simulink model "simDron"  (R2024a)
settings: Solver=VariableStepAuto  StartTime=0.0  StopTime=t  RelTol=1e-6  AbsTol=1e-9
values from neighbouring files (symbols this model uses):
  d0 = [0;0;-2]    [Dron.m]
  I = [Ixx, 0, 0 ... (first row only)    [Dron.m]
  Jr = -5.897e-8    (= -5.897e-08)    [Dron.m]
  km = 803.9    [Dron.m]
  KQ = 1.058e-10    [Dron.m]
  KT = 3.334e-8    (= 3.334e-08)    [Dron.m]
  l = 0.058    [Dron.m]
  m = 0.045    [Dron.m]
  mg = [0;0;m*9.81]    [Dron.m]
  theta0 = [0;0;0]    [Dron.m]
  u1 = 10000    [Dron.m]
  u2 = 5000    [Dron.m]
  u3 = 10000    [Dron.m]
  u4 = 5000    [Dron.m]
  v0 = [0;0;0]    [Dron.m]
  w0 = [0;0;0]    [Dron.m]
libraries: matrix_library x2
settings Model: Creator=oscka  LastModifiedBy=oscka
settings DataIOCC: SaveOutput=off  SignalLogging=off  DSMLogging=off  SaveTime=off  ReturnWorkspaceOutputs=off

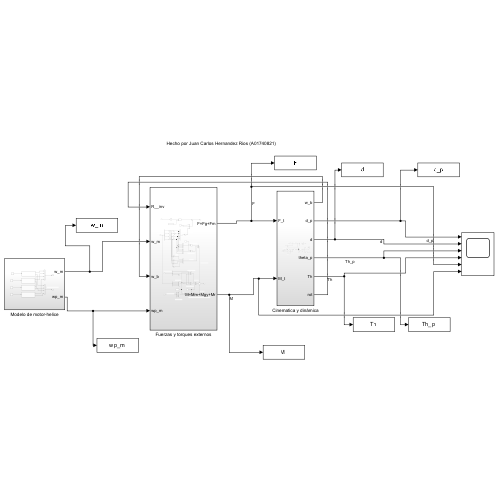
[thumbnail: Simulink's stored preview of the top-level diagram]
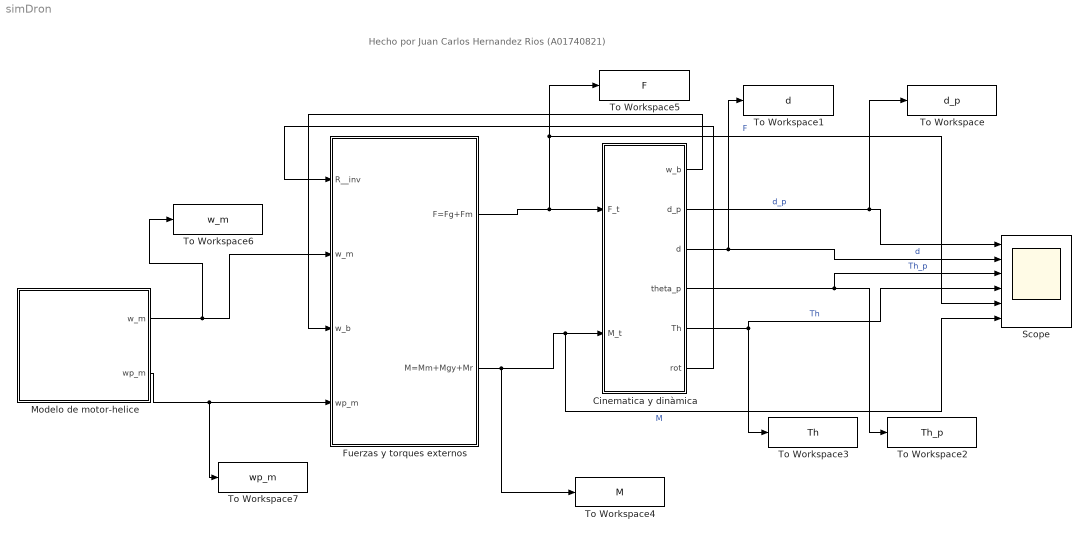
== system simDron ==
  note: Hecho por Juan Carlos Hernandez Rios (A01740821)
  Cinematica y dinàmica : Subsystem
  Fuerzas y torques externos : Subsystem
  Modelo de motor-helice : Subsystem
  Scope : Scope  NumInputPorts=6
  To Workspace : ToWorkspace  VariableName=d_p  SaveFormat=Timeseries  SampleTime=-1
  To Workspace1 : ToWorkspace  VariableName=d  SaveFormat=Timeseries  SampleTime=-1
  To Workspace2 : ToWorkspace  VariableName=Th_p  SaveFormat=Timeseries  SampleTime=-1
  To Workspace3 : ToWorkspace  VariableName=Th  SaveFormat=Timeseries  SampleTime=-1
  To Workspace4 : ToWorkspace  VariableName=M  SaveFormat=Timeseries  SampleTime=-1
  To Workspace5 : ToWorkspace  VariableName=F  SaveFormat=Timeseries  SampleTime=-1
  To Workspace6 : ToWorkspace  VariableName=w_m  SaveFormat=Timeseries  SampleTime=-1
  To Workspace7 : ToWorkspace  VariableName=wp_m  SaveFormat=Timeseries  SampleTime=-1
  wires:
  Modelo de motor-helice/1(w_m) -> To Workspace6/1, Fuerzas y torques externos/2(w_m)
  Modelo de motor-helice/2(wp_m) -> To Workspace7/1, Fuerzas y torques externos/4(wp_m)
  Fuerzas y torques externos/1(F=Fg+Fm) -> To Workspace5/1, Scope/5, Cinematica y dinàmica/1(F_t)  "F"
  Fuerzas y torques externos/2(M=Mm+Mgy+Mr) -> Scope/6, Cinematica y dinàmica/2(M_t), To Workspace4/1  "M"
  Cinematica y dinàmica/1(w_b) -> Fuerzas y torques externos/3(w_b)
  Cinematica y dinàmica/6(rot) -> Fuerzas y torques externos/1(R__inv)
  Cinematica y dinàmica/2(d_p) -> To Workspace/1, Scope/1  "d_p"
  Cinematica y dinàmica/3(d) -> Scope/2, To Workspace1/1  "d"
  Cinematica y dinàmica/4(theta_p) -> Scope/3, To Workspace2/1  "Th_p"
  Cinematica y dinàmica/5(Th) -> Scope/4, To Workspace3/1  "Th"

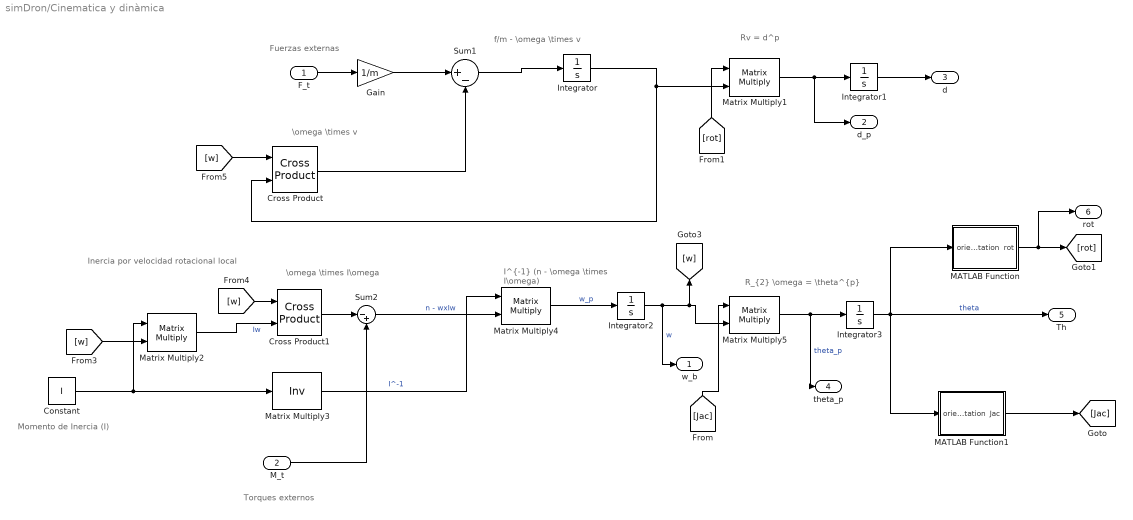
== system simDron/Cinematica y dinàmica ==
  note: Fuerzas externas
  note: Torques externos
  note: Rv = d^p
  note: \omega \times v
  note: f/m - \omega \times v
  note: I^{-1} (n - \omega \times I\omega)
  note: R_{2} \omega = \theta^{p}
  note: \omega \times I\omega
  note: Momento de Inercia (I)
  note: Inercia por velocidad rotacional local
  F_t : Inport
  M_t : Inport  Port=2
  Constant : Constant  Value=I  VectorParams1D=off
  Cross Product : matrix_library/Cross Product
  Cross Product1 : matrix_library/Cross Product
  Gain : Gain  Gain=1/m
  Integrator : Integrator  InitialCondition=v0
  Integrator1 : Integrator  InitialCondition=d0
  Integrator2 : Integrator  InitialCondition=w0
  Integrator3 : Integrator  InitialCondition=theta0
  MATLAB Function : MATLAB Function  TreatAsAtomicUnit=on
  MATLAB Function1 : MATLAB Function  TreatAsAtomicUnit=on
  Matrix Multiply{1..2,4..5} (4 alike) : Product  Multiplication=Matrix(*)
  Matrix Multiply3 : Product  Inputs=/  Multiplication=Matrix(*)
  Sum1 : Sum  Inputs=|+-
  Sum2 : Sum  Inputs=|-+
  w_b : Outport
  d_p : Outport  Port=2
  d : Outport  Port=3
  theta_p : Outport  Port=4
  Th : Outport  Port=5
  rot : Outport  Port=6
  wires:
  [Jac] -> Matrix Multiply5/1
  Matrix Multiply2/1 -> Cross Product1/2  "Iw"
  [w] -> Cross Product1/1
  [w] -> Matrix Multiply2/2
  MATLAB Function1/1(Jac) -> [Jac]
  Matrix Multiply1/1 -> d_p/1, Integrator1/1
  [w] -> Cross Product/1
  Matrix Multiply5/1 -> theta_p/1, Integrator3/1  "theta_p"
  Integrator2/1 -> w_b/1, [w], Matrix Multiply5/2  "w"
  Cross Product/1 -> Sum1/2
  Cross Product1/1 -> Sum2/1
  MATLAB Function/1(rot) -> rot/1, [rot]
  Matrix Multiply3/1 -> Matrix Multiply4/1  "I^-1"
  Matrix Multiply4/1 -> Integrator2/1  "w_p"
  Integrator3/1 -> MATLAB Function/1(orientation), MATLAB Function1/1(orientation), Th/1  "theta"
  Sum2/1 -> Matrix Multiply4/2  "n - wxIw"
  Constant/1 -> Matrix Multiply2/1, Matrix Multiply3/1
  Integrator/1 -> Matrix Multiply1/2, Cross Product/2
  [rot] -> Matrix Multiply1/1
  Sum1/1 -> Integrator/1
  Integrator1/1 -> d/1
  M_t/1 -> Sum2/2
  Gain/1 -> Sum1/1
  F_t/1 -> Gain/1

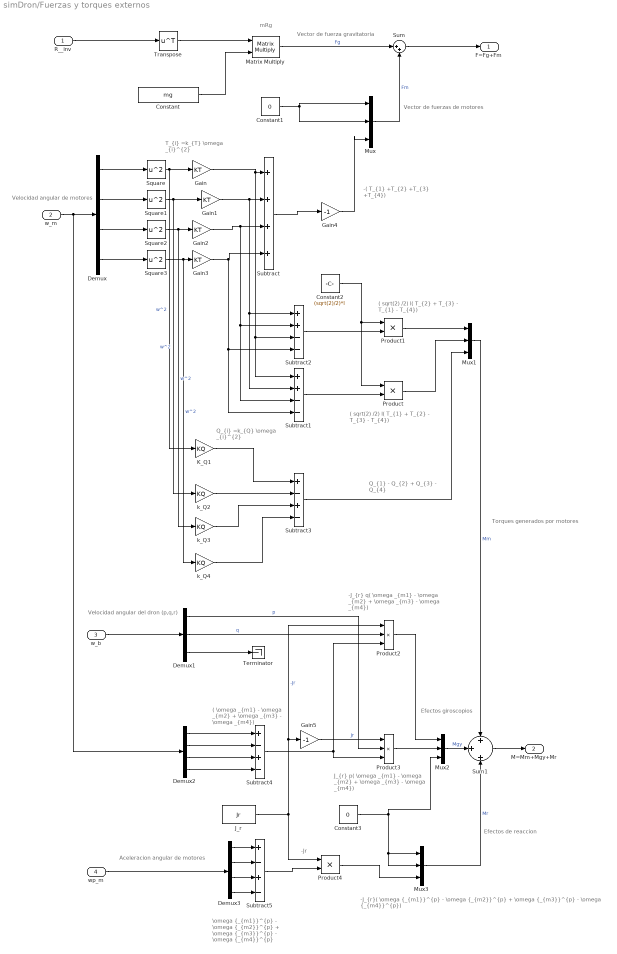
== system simDron/Fuerzas y torques externos ==
  note: \omega {_{m1}}^{p} - \omega {_{m2}}^{p} + \omega {_{m3}}^{p} - \omega {_{m4}}^{p}
  note: ( \omega _{m1} - \omega _{m2} + \omega _{m3} - \omega _{m4})
  note: Velocidad angular de motores
  note: Velocidad angular del dron (p,q,r)
  note: Aceleracion angular de motores
  note: -J_{r}( \omega {_{m1}}^{p} - \omega {_{m2}}^{p} + \omega {_{m3}}^{p} - \omega {_{m4}}^{p})
  note: -Jr
  note: J_{r} p( \omega _{m1} - \omega _{m2} + \omega _{m3} - \omega _{m4})
  note: -J_{r} q( \omega _{m1} - \omega _{m2} + \omega _{m3} - \omega _{m4})
  note: Efectos de reaccion
  note: Efectos giroscopios
  note: Torques generados por motores
  note: ( sqrt(2) /2) l( T_{2} + T_{3} - T_{1} - T_{4})
  note: Q_{1} - Q_{2} + Q_{3} - Q_{4}
  note: Q_{i} =k_{Q} \omega _{i}^{2}
  note: T_{i} =k_{T} \omega _{i}^{2}
  note: Vector de fuerza gravitatoria
  note: Vector de fuerzas de motores
  note: -( T_{1} +T_{2} +T_{3} +T_{4})
  note: mRg
  note: ( sqrt(2) /2) l( T_{1} + T_{2} - T_{3} - T_{4})
  R__inv : Inport
  w_m : Inport  Port=2
  w_b : Inport  Port=3
  wp_m : Inport  Port=4
  Constant : Constant  Value=mg
  Constant1 : Constant  Value=0
  Constant2 : Constant  Value=(sqrt(2)/2)*l
  Constant3 : Constant  Value=0
  Demux : Demux
  Demux1 : Demux  Outputs=3
  Demux2 : Demux
  Demux3 : Demux
  Gain{,1..3} (4 alike) : Gain  Gain=KT
  Gain4 : Gain  Gain=-1
  Gain5 : Gain  Gain=-1
  J_r : Constant  Value=Jr
  K_Q1 : Gain  Gain=KQ
  Matrix Multiply : Product  Multiplication=Matrix(*)
  Mux{,1..3} (4 alike) : Mux  Inputs=3
  Product : Product
  Product1 : Product
  Product2 : Product  Inputs=3
  Product3 : Product  Inputs=3
  Product4 : Product
  Square{,1..3} (4 alike) : Math  Operator=square
  Subtract : Sum  Inputs=++++
  Subtract1 : Sum  Inputs=++--
  Subtract2 : Sum  Inputs=++--
  Subtract3 : Sum  Inputs=+-+-
  Subtract4 : Sum  Inputs=+-+-
  Subtract5 : Sum  Inputs=+-+-
  Sum : Sum  Inputs=|++
  Sum1 : Sum  Inputs=+|+|+
  Terminator : Terminator
  Transpose : Math  Operator=transpose
  k_Q2 : Gain  Gain=KQ
  k_Q3 : Gain  Gain=KQ
  k_Q4 : Gain  Gain=KQ
  F=Fg+Fm : Outport
  M=Mm+Mgy+Mr : Outport  Port=2
  wires:
  Gain3/1 -> Subtract2/4, Subtract1/4, Subtract/4
  Transpose/1 -> Matrix Multiply/1
  Gain/1 -> Subtract2/3, Subtract1/1, Subtract/1
  Subtract/1 -> Gain4/1
  Sum/1 -> F=Fg+Fm/1
  Constant1/1 -> Mux/2, Mux/1
  w_m/1 -> Demux2/1, Demux/1
  Gain4/1 -> Mux/3
  Gain2/1 -> Subtract2/2, Subtract1/3, Subtract/3
  Square3/1 -> k_Q4/1, Gain3/1  "w^2"
  Demux/3 -> Square2/1
  Constant/1 -> Matrix Multiply/2
  Gain1/1 -> Subtract2/1, Subtract1/2, Subtract/2
  Mux/1 -> Sum/2  "Fm"
  Square2/1 -> k_Q3/1, Gain2/1  "w^2"
  R__inv/1 -> Transpose/1
  Demux/4 -> Square3/1
  Square1/1 -> k_Q2/1, Gain1/1  "w^2"
  Square/1 -> K_Q1/1, Gain/1  "w^2"
  Demux/2 -> Square1/1
  Demux/1 -> Square/1
  Matrix Multiply/1 -> Sum/1  "Fg"
  Constant2/1 -> Product1/1, Product/1
  Subtract1/1 -> Product/2
  Subtract2/1 -> Product1/2
  Product1/1 -> Mux1/1
  Product/1 -> Mux1/2
  K_Q1/1 -> Subtract3/1
  k_Q2/1 -> Subtract3/2
  k_Q3/1 -> Subtract3/3
  k_Q4/1 -> Subtract3/4
  Subtract3/1 -> Mux1/3
  w_b/1 -> Demux1/1
  Demux1/3 -> Terminator/1
  Demux1/2 -> Product2/2  "q"
  Demux2/1 -> Subtract4/1
  Demux2/2 -> Subtract4/2
  Demux2/3 -> Subtract4/3
  Demux2/4 -> Subtract4/4
  Subtract4/1 -> Product2/3, Product3/3
  J_r/1 -> Product2/1, Gain5/1, Product4/1  "-Jr"
  Demux1/1 -> Product3/2  "p"
  Gain5/1 -> Product3/1  "Jr"
  wp_m/1 -> Demux3/1
  Demux3/1 -> Subtract5/1
  Demux3/2 -> Subtract5/2
  Demux3/3 -> Subtract5/3
  Demux3/4 -> Subtract5/4
  Subtract5/1 -> Product4/2
  Product4/1 -> Mux3/3
  Constant3/1 -> Mux2/3, Mux3/2, Mux3/1
  Product3/1 -> Mux2/2
  Product2/1 -> Mux2/1
  Mux2/1 -> Sum1/2  "Mgy"
  Mux3/1 -> Sum1/3  "Mr"
  Mux1/1 -> Sum1/1  "Mm"
  Sum1/1 -> M=Mm+Mgy+Mr/1

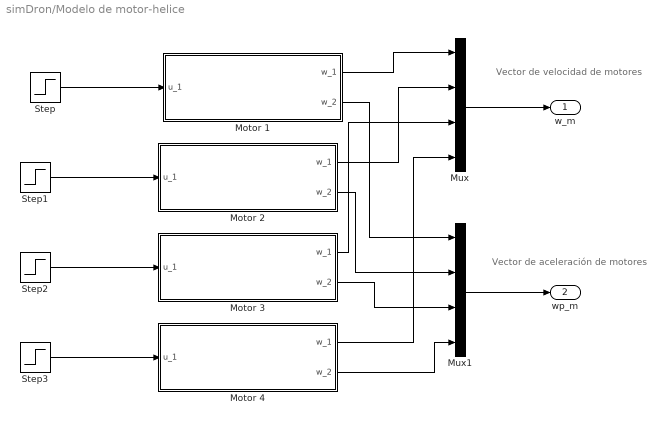
== system simDron/Modelo de motor-helice ==
  note: Vector de aceleración de motores
  note: Vector de velocidad de motores
  Motor 1 : Subsystem
  Motor 2 : Subsystem
  Motor 3 : Subsystem
  Motor 4 : Subsystem
  Mux : Mux
  Mux1 : Mux
  Step : Step  Time=0.1  After=u1  SampleTime=0.1  VectorParams1D=off
  Step1 : Step  Time=0.1  After=u2  SampleTime=0.1  VectorParams1D=off
  Step2 : Step  Time=0.1  After=u3  SampleTime=0.1  VectorParams1D=off
  Step3 : Step  Time=0.1  After=u4  SampleTime=0.1  VectorParams1D=off
  w_m : Outport
  wp_m : Outport  Port=2
  wires:
  Motor 3/2(w_2) -> Mux1/3
  Mux1/1 -> wp_m/1
  Motor 4/1(w_1) -> Mux/4
  Mux/1 -> w_m/1
  Motor 2/2(w_2) -> Mux1/2
  Motor 1/2(w_2) -> Mux1/1
  Motor 1/1(w_1) -> Mux/1
  Motor 3/1(w_1) -> Mux/3
  Motor 2/1(w_1) -> Mux/2
  Motor 4/2(w_2) -> Mux1/4
  Step/1 -> Motor 1/1(u_1)
  Step1/1 -> Motor 2/1(u_1)
  Step2/1 -> Motor 3/1(u_1)
  Step3/1 -> Motor 4/1(u_1)

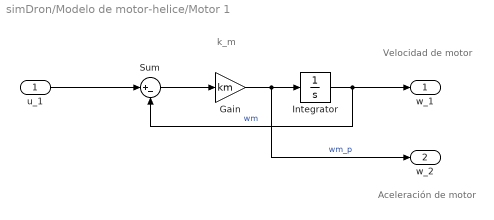
== system simDron/Modelo de motor-helice/Motor 1 ==
  note: Velocidad de motor
  note: k_m
  note: Aceleración de motor
  u_1 : Inport
  Gain : Gain  Gain=km
  Integrator : Integrator
  Sum : Sum  Inputs=|+-
  w_1 : Outport
  w_2 : Outport  Port=2
  wires:
  Integrator/1 -> w_1/1, Sum/2  "wm"
  Sum/1 -> Gain/1
  u_1/1 -> Sum/1
  Gain/1 -> w_2/1, Integrator/1  "wm_p"

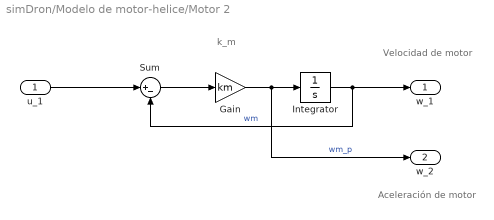
== system simDron/Modelo de motor-helice/Motor 2 ==
  note: Velocidad de motor
  note: k_m
  note: Aceleración de motor
  u_1 : Inport
  Gain : Gain  Gain=km
  Integrator : Integrator
  Sum : Sum  Inputs=|+-
  w_1 : Outport
  w_2 : Outport  Port=2
  wires:
  Integrator/1 -> w_1/1, Sum/2  "wm"
  Sum/1 -> Gain/1
  u_1/1 -> Sum/1
  Gain/1 -> w_2/1, Integrator/1  "wm_p"

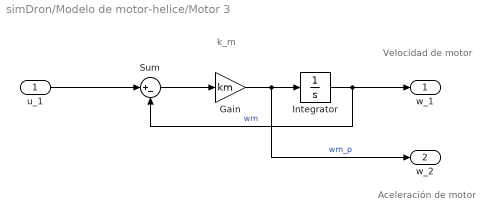
== system simDron/Modelo de motor-helice/Motor 3 ==
  note: Velocidad de motor
  note: k_m
  note: Aceleración de motor
  u_1 : Inport
  Gain : Gain  Gain=km
  Integrator : Integrator
  Sum : Sum  Inputs=|+-
  w_1 : Outport
  w_2 : Outport  Port=2
  wires:
  Integrator/1 -> w_1/1, Sum/2  "wm"
  Sum/1 -> Gain/1
  u_1/1 -> Sum/1
  Gain/1 -> w_2/1, Integrator/1  "wm_p"

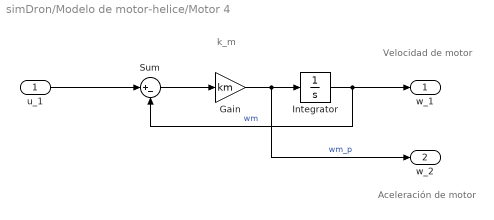
== system simDron/Modelo de motor-helice/Motor 4 ==
  note: Velocidad de motor
  note: k_m
  note: Aceleración de motor
  u_1 : Inport
  Gain : Gain  Gain=km
  Integrator : Integrator
  Sum : Sum  Inputs=|+-
  w_1 : Outport
  w_2 : Outport  Port=2
  wires:
  Integrator/1 -> w_1/1, Sum/2  "wm"
  Sum/1 -> Gain/1
  u_1/1 -> Sum/1
  Gain/1 -> w_2/1, Integrator/1  "wm_p"

== matlab function simDron/Cinematica y dinàmica/MATLAB Function ==
  data: orientation input; rot output
function rot = fcn(orientation)

phi = orientation(1)
theta = orientation(2);
psi = orientation(3);

rot = [cos(theta)*cos(psi), cos(theta)*sin(psi), -sin(theta);
       -cos(phi)*sin(psi)+sin(phi)*sin(theta)*cos(psi), cos(phi)*cos(psi)+sin(phi)*sin(theta)*sin(psi), sin(phi)*cos(theta);
       sin(phi)*sin(psi)+cos(phi)*sin(theta)*cos(psi), -sin(phi)*cos(psi)+cos(phi)*sin(theta)*sin(psi), cos(phi)*cos(theta)];

rot = rot';

== matlab function simDron/Cinematica y dinàmica/MATLAB Function1 ==
  data: orientation input; Jac output
function Jac = fcn(orientation)

phi = orientation(1);
theta = orientation(2);
psi = orientation(3);

Jac = [1, sin(phi)*tan(theta), cos(phi)*tan(theta);
       0, cos(phi),            -sin(phi);
       0, sin(phi)/cos(theta), cos(phi)/cos(theta)];
